simulink model "Quadcopter_nonlinear_LQR"  (R2020a)
settings: Solver=ode4  StartTime=0.0  StopTime=15  FixedStep=0.01  RelTol=1e-3
InitFcn:
  | linear_LQR_riccati_solver
values from neighbouring files (symbols this model uses):
  A1 = (h_cg * g * m_tot) / (m_tot * h_cg^2 + J_xx)    [QuadConstants.m]
  A2 = (2*m_tot * h_cg^2 + J_yy -J_zz) / (m_tot * h_cg^2 + J_xx)    [QuadConstants.m]
  A3 = (b * d_cg) / (m_tot * h_cg^2 + J_xx)    [QuadConstants.m]
  A4 = (J_R) / (m_tot * h_cg^2 + J_xx)    [QuadConstants.m]
  A5 = (m1 * g * miu_k * r_x) / (m_tot * h_cg^2 + J_xx)    [QuadConstants.m]
  B1 = (h_cg * g * m_tot) / (m_tot * h_cg^2 + J_yy)    [QuadConstants.m]
  B2 = (-2*m_tot * h_cg^2 - J_xx + J_zz) / (m_tot * h_cg^2 + J_yy)    [QuadConstants.m]
  B3 = (b * d_cg) / (m_tot * h_cg^2 + J_yy)    [QuadConstants.m]
  B4 = (-J_R) / (m_tot * h_cg^2 + J_yy)    [QuadConstants.m]
  B5 = (m2 * g * miu_k * r_y) / (m_tot * h_cg^2 + J_yy)    [QuadConstants.m]
  C1 = (J_xx - J_yy) / (J_zz)    [QuadConstants.m]
  C2 = (d) / (J_zz)    [QuadConstants.m]
  C3 = (m3 * g * miu_k * r_z) / (J_zz)    [QuadConstants.m]
undefined symbols (not defined in the file or in its folder): LQR_feedback_gain, magnitude, x0
settings Model: Creator=Ali  LastModifiedBy=Ali

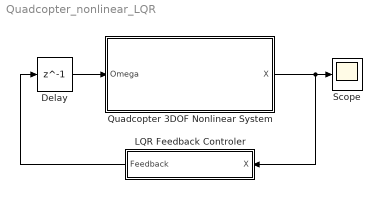
== system Quadcopter_nonlinear_LQR ==
  Delay : Delay  DelayLength=1
  LQR Feedback Controler : Subsystem
  Quadcopter 3DOF Nonlinear System : Subsystem  TreatAsAtomicUnit=on
  Scope : Scope
  wires:
  Quadcopter 3DOF Nonlinear System/1(X) -> LQR Feedback Controler/1(X), Scope/1
  LQR Feedback Controler/1(Feedback) -> Delay/1
  Delay/1 -> Quadcopter 3DOF Nonlinear System/1(Omega)

== system Quadcopter_nonlinear_LQR/LQR Feedback Controler ==
  X : Inport
  Add : Sum
  Constant : Constant  Value=LQR_feedback_gain
  Constant1 : Constant  Value=2000
  Product : Product  Multiplication=Matrix(*)
  Feedback : Outport
  wires:
  X/1 -> Product/2
  Constant/1 -> Product/1
  Product/1 -> Add/2
  Constant1/1 -> Add/1
  Add/1 -> Feedback/1

== system Quadcopter_nonlinear_LQR/Quadcopter 3DOF Nonlinear System ==
  Omega : Inport
  Integrator : Integrator  InitialCondition=x0
  Quad System : Subsystem
  X : Outport
  wires:
  Integrator/1 -> Quad System/1(X), X/1  "X"
  Quad System/1(dot(X)) -> Integrator/1  "dot(X)"
  Omega/1 -> Quad System/2(Omega)

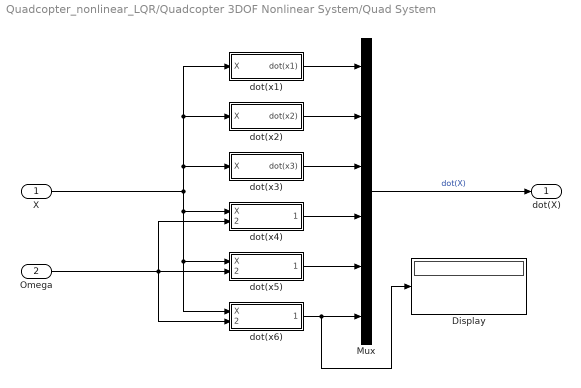
== system Quadcopter_nonlinear_LQR/Quadcopter 3DOF Nonlinear System/Quad System ==
  X : Inport
  Omega : Inport  Port=2
  Display : Display
  Mux : Mux  Inputs=6
  dot(x1) : Subsystem
  dot(x2) : Subsystem
  dot(x3) : Subsystem
  dot(x4) : Subsystem
  dot(x5) : Subsystem
  dot(x6) : Subsystem
  dot(X) : Outport
  wires:
  Mux/1 -> dot(X)/1  "dot(X)"
  X/1 -> dot(x1)/1(X), dot(x2)/1(X), dot(x3)/1(X), dot(x6)/1(X), dot(x5)/1(X), dot(x4)/1(X)
  Omega/1 -> dot(x4)/2(Omega), dot(x6)/2(Omega), dot(x5)/2(Omega)
  dot(x5)/1(dot(x5)) -> Mux/5
  dot(x2)/1(dot(x2)) -> Mux/2
  dot(x4)/1(dot(x4)) -> Mux/4
  dot(x3)/1(dot(x3)) -> Mux/3
  dot(x1)/1(dot(x1)) -> Mux/1
  dot(x6)/1(dot(x6)) -> Display/1, Mux/6

== system Quadcopter_nonlinear_LQR/Quadcopter 3DOF Nonlinear System/Quad System/dot(x1) ==
  X : Inport
  1 : Subsystem
  Add : Sum  Inputs=+++
  Subsystem : Subsystem
  Subsystem1 : Subsystem
  dot(x1) : Outport
  wires:
  X/1 -> Subsystem1/1(X), Subsystem/1(X), 1/1(X)  "X"
  Subsystem1/1(x4) -> Add/3
  Subsystem/1(x6cos(x1)tan(x2)) -> Add/2
  Add/1 -> dot(x1)/1
  1/1(x5sin(x1)tan(x2)) -> Add/1

== system Quadcopter_nonlinear_LQR/Quadcopter 3DOF Nonlinear System/Quad System/dot(x2) ==
  X : Inport
  1 : Subsystem
  Add : Sum  Inputs=+-
  Subsystem : Subsystem
  dot(x2) : Outport
  wires:
  X/1 -> 1/1(X), Subsystem/1(X)  "X"
  Subsystem/1(x6sin(x1)) -> Add/2
  Add/1 -> dot(x2)/1
  1/1(x5cos(x1)) -> Add/1

== system Quadcopter_nonlinear_LQR/Quadcopter 3DOF Nonlinear System/Quad System/dot(x3) ==
  X : Inport
  1 : Subsystem
  Add : Sum
  Product : Product
  Subsystem : Subsystem
  Subsystem1 : Subsystem
  dot(x3) : Outport
  wires:
  X/1 -> Subsystem1/1(X), Subsystem/1(X), 1/1(X)  "X"
  Subsystem/1(x6cos(x1)) -> Add/2
  1/1(x5sin(x1)) -> Add/1
  Product/1 -> dot(x3)/1
  Add/1 -> Product/1
  Subsystem1/1(sec(x2)) -> Product/2

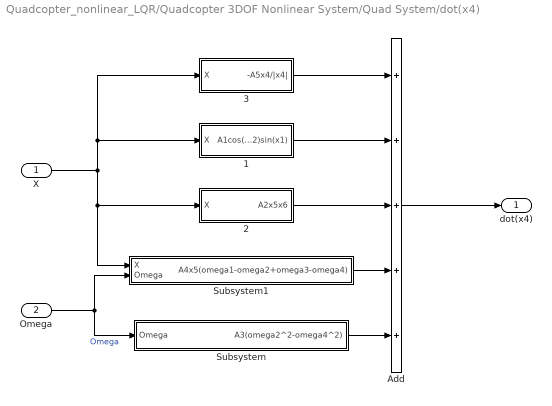
== system Quadcopter_nonlinear_LQR/Quadcopter 3DOF Nonlinear System/Quad System/dot(x4) ==
  X : Inport
  Omega : Inport  Port=2
  1 : Subsystem
  2 : Subsystem
  3 : Subsystem
  Add : Sum  Inputs=+++++
  Subsystem : Subsystem
  Subsystem1 : Subsystem
  dot(x4) : Outport
  wires:
  X/1 -> Subsystem1/1(X), 2/1(X), 3/1(X), 1/1(X)
  Omega/1 -> Subsystem1/2(Omega), Subsystem/1(Omega)  "Omega"
  Add/1 -> dot(x4)/1
  3/1("-A5x4/|x4| ") -> Add/1
  1/1(A1cos(x2)sin(x1)) -> Add/2
  2/1(A2x5x6) -> Add/3
  Subsystem1/1(A4x5(omega1-omega2+omega3-omega4)) -> Add/4
  Subsystem/1(A3(omega2^2-omega4^2)) -> Add/5

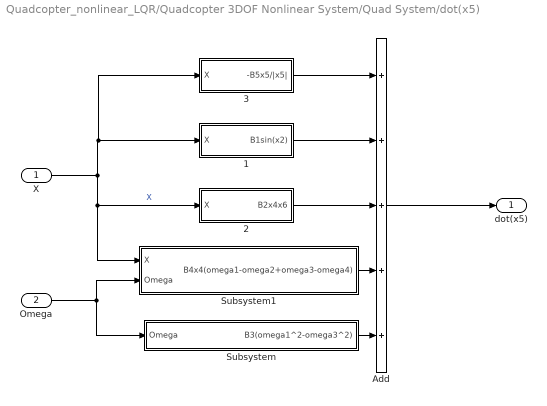
== system Quadcopter_nonlinear_LQR/Quadcopter 3DOF Nonlinear System/Quad System/dot(x5) ==
  X : Inport
  Omega : Inport  Port=2
  1 : Subsystem
  2 : Subsystem
  3 : Subsystem
  Add : Sum  Inputs=+++++
  Subsystem : Subsystem
  Subsystem1 : Subsystem
  dot(x5) : Outport
  wires:
  X/1 -> Subsystem1/1(X), 2/1(X), 3/1(X), 1/1(X)  "X"
  Omega/1 -> Subsystem/1(Omega), Subsystem1/2(Omega)
  Add/1 -> dot(x5)/1
  3/1("-B5x5/|x5| ") -> Add/1
  1/1(B1sin(x2)) -> Add/2
  2/1(B2x4x6) -> Add/3
  Subsystem1/1(B4x4(omega1-omega2+omega3-omega4)) -> Add/4
  Subsystem/1(B3(omega1^2-omega3^2)) -> Add/5

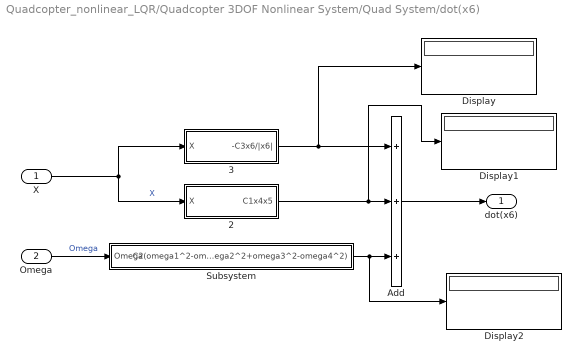
== system Quadcopter_nonlinear_LQR/Quadcopter 3DOF Nonlinear System/Quad System/dot(x6) ==
  X : Inport
  Omega : Inport  Port=2
  2 : Subsystem
  3 : Subsystem
  Add : Sum  Inputs=+++
  Display : Display
  Display1 : Display
  Display2 : Display
  Subsystem : Subsystem
  dot(x6) : Outport
  wires:
  Omega/1 -> Subsystem/1(Omega)  "Omega"
  Add/1 -> dot(x6)/1
  3/1("-C3x6/|x6| ") -> Display/1, Add/1
  2/1(C1x4x5) -> Display1/1, Add/2
  Subsystem/1(C2(omega1^2-omega2^2+omega3^2-omega4^2)) -> Display2/1, Add/3
  X/1 -> 3/1(X), 2/1(X)  "X"

== system Quadcopter_nonlinear_LQR/Quadcopter 3DOF Nonlinear System/Quad System/dot(x1)/1 ==
  X : Inport
  Demux : Demux  Outputs=6
  Subsystem : Subsystem
  Terminator : Terminator
  Terminator1 : Terminator
  Terminator2 : Terminator
  x5sin(x1)tan(x2) : Outport
  wires:
  Demux/2 -> Subsystem/2(x2)  "x2"
  Demux/4 -> Terminator1/1  "x4"
  X/1 -> Demux/1  "x"
  Demux/1 -> Subsystem/1(x1)  "x1"
  Demux/3 -> Terminator/1  "x3"
  Demux/6 -> Terminator2/1  "x6"
  Demux/5 -> Subsystem/3(x5)  "x5"
  Subsystem/1(x5sin(x1)tan(x2)) -> x5sin(x1)tan(x2)/1

== system Quadcopter_nonlinear_LQR/Quadcopter 3DOF Nonlinear System/Quad System/dot(x1)/Subsystem ==
  X : Inport
  Demux : Demux  Outputs=6
  Subsystem1 : Subsystem
  Terminator : Terminator
  Terminator1 : Terminator
  Terminator3 : Terminator
  x6cos(x1)tan(x2) : Outport
  wires:
  Demux/1 -> Subsystem1/1(x1)  "x1"
  Demux/3 -> Terminator/1  "x3"
  Demux/4 -> Terminator1/1  "x4"
  Demux/5 -> Terminator3/1  "x5"
  Demux/6 -> Subsystem1/3(x6)  "x6"
  Subsystem1/1(x6cos(x1)tan(x2)) -> x6cos(x1)tan(x2)/1  "x6cos(x1)tan(x2)"
  X/1 -> Demux/1  "X"
  Demux/2 -> Subsystem1/2(x2)  "x2"

== system Quadcopter_nonlinear_LQR/Quadcopter 3DOF Nonlinear System/Quad System/dot(x1)/Subsystem1 ==
  X : Inport
  Demux : Demux  Outputs=6
  Terminator{,2..5} (5 alike) : Terminator
  x4 : Outport
  wires:
  Demux/6 -> Terminator5/1  "x6"
  X/1 -> Demux/1
  Demux/3 -> Terminator/1  "x3"
  Demux/1 -> Terminator4/1  "x1"
  Demux/2 -> Terminator2/1  "x2"
  Demux/5 -> Terminator3/1  "x5"
  Demux/4 -> x4/1  "x4"

== system Quadcopter_nonlinear_LQR/Quadcopter 3DOF Nonlinear System/Quad System/dot(x2)/1 ==
  X : Inport
  Demux : Demux  Outputs=6
  Subsystem : Subsystem
  Terminator{,1..3} (4 alike) : Terminator
  x5cos(x1) : Outport
  wires:
  Demux/4 -> Terminator1/1  "x4"
  X/1 -> Demux/1  "x"
  Demux/1 -> Subsystem/1(x1)  "x1"
  Demux/3 -> Terminator/1  "x3"
  Demux/6 -> Terminator2/1  "x6"
  Demux/5 -> Subsystem/2(x5)  "x5"
  Subsystem/1(Out1) -> x5cos(x1)/1
  Demux/2 -> Terminator3/1  "x2"

== system Quadcopter_nonlinear_LQR/Quadcopter 3DOF Nonlinear System/Quad System/dot(x2)/Subsystem ==
  X : Inport
  Demux : Demux  Outputs=6
  Subsystem1 : Subsystem
  Terminator{,1..3} (4 alike) : Terminator
  x6sin(x1) : Outport
  wires:
  Demux/1 -> Subsystem1/1(x1)  "x1"
  Demux/3 -> Terminator/1  "x3"
  Demux/4 -> Terminator1/1  "x4"
  Demux/5 -> Terminator3/1  "x5"
  Demux/6 -> Subsystem1/2(x6)  "x6"
  Subsystem1/1(Out1) -> x6sin(x1)/1  "x6sin(x1)"
  X/1 -> Demux/1  "X"
  Demux/2 -> Terminator2/1  "x2"

== system Quadcopter_nonlinear_LQR/Quadcopter 3DOF Nonlinear System/Quad System/dot(x3)/1 ==
  X : Inport
  Demux : Demux  Outputs=6
  Subsystem : Subsystem
  Terminator{,1..3} (4 alike) : Terminator
  x5sin(x1) : Outport
  wires:
  Demux/4 -> Terminator1/1  "x4"
  X/1 -> Demux/1  "x"
  Demux/1 -> Subsystem/1(x1)  "x1"
  Demux/3 -> Terminator/1  "x3"
  Demux/6 -> Terminator2/1  "x6"
  Demux/5 -> Subsystem/2(x5)  "x5"
  Subsystem/1(x5sin(x1)) -> x5sin(x1)/1
  Demux/2 -> Terminator3/1  "x2"

== system Quadcopter_nonlinear_LQR/Quadcopter 3DOF Nonlinear System/Quad System/dot(x3)/Subsystem ==
  X : Inport
  Demux : Demux  Outputs=6
  Subsystem1 : Subsystem
  Terminator{,1..3} (4 alike) : Terminator
  x6cos(x1) : Outport
  wires:
  Demux/1 -> Subsystem1/1(x1)  "x1"
  Demux/3 -> Terminator/1  "x3"
  Demux/4 -> Terminator1/1  "x4"
  Demux/5 -> Terminator3/1  "x5"
  Demux/6 -> Subsystem1/2(x6)  "x6"
  Subsystem1/1(Out1) -> x6cos(x1)/1  "x6cos(x1)"
  X/1 -> Demux/1  "X"
  Demux/2 -> Terminator2/1  "x2"

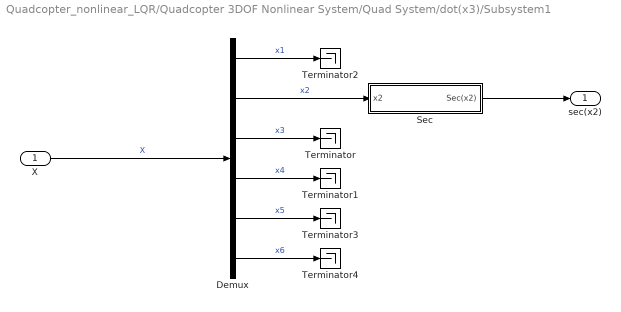
== system Quadcopter_nonlinear_LQR/Quadcopter 3DOF Nonlinear System/Quad System/dot(x3)/Subsystem1 ==
  X : Inport
  Demux : Demux  Outputs=6
  Sec : Subsystem
  Terminator{,1..4} (5 alike) : Terminator
  sec(x2) : Outport
  wires:
  Demux/3 -> Terminator/1  "x3"
  Demux/4 -> Terminator1/1  "x4"
  Demux/5 -> Terminator3/1  "x5"
  X/1 -> Demux/1  "X"
  Demux/1 -> Terminator2/1  "x1"
  Demux/6 -> Terminator4/1  "x6"
  Demux/2 -> Sec/1(x2)  "x2"
  Sec/1(Sec(x2)) -> sec(x2)/1

== system Quadcopter_nonlinear_LQR/Quadcopter 3DOF Nonlinear System/Quad System/dot(x4)/1 ==
  X : Inport
  Demux : Demux  Outputs=6
  Subsystem : Subsystem
  Terminator{,1..3} (4 alike) : Terminator
  A1cos(x2)sin(x1) : Outport
  wires:
  Demux/4 -> Terminator1/1  "x4"
  X/1 -> Demux/1  "x"
  Demux/1 -> Subsystem/1(x1)  "x1"
  Demux/3 -> Terminator/1  "x3"
  Demux/6 -> Terminator2/1  "x6"
  Subsystem/1(A1cos(x2)sin(x1)) -> A1cos(x2)sin(x1)/1
  Demux/2 -> Subsystem/2(x2)  "x2"
  Demux/5 -> Terminator3/1  "x5"

== system Quadcopter_nonlinear_LQR/Quadcopter 3DOF Nonlinear System/Quad System/dot(x4)/2 ==
  X : Inport
  Demux : Demux  Outputs=6
  Subsystem : Subsystem
  Terminator{,1,4..5} (4 alike) : Terminator
  A2x5x6 : Outport
  wires:
  Demux/4 -> Terminator1/1  "x4"
  X/1 -> Demux/1  "x"
  Demux/3 -> Terminator/1  "x3"
  Demux/6 -> Subsystem/2(x6)  "x6"
  Subsystem/1(A2x5x6) -> A2x5x6/1
  Demux/5 -> Subsystem/1(x5)  "x5"
  Demux/1 -> Terminator4/1  "x1"
  Demux/2 -> Terminator5/1  "x2"

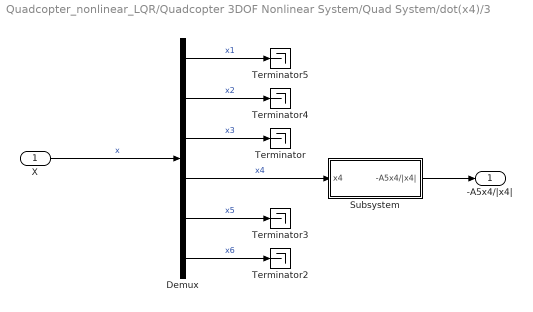
== system Quadcopter_nonlinear_LQR/Quadcopter 3DOF Nonlinear System/Quad System/dot(x4)/3 ==
  X : Inport
  Demux : Demux  Outputs=6
  Subsystem : Subsystem
  Terminator{,2..5} (5 alike) : Terminator
  "-A5x4/|x4| " : Outport
  wires:
  X/1 -> Demux/1  "x"
  Demux/1 -> Terminator5/1  "x1"
  Demux/3 -> Terminator/1  "x3"
  Demux/6 -> Terminator2/1  "x6"
  Demux/2 -> Terminator4/1  "x2"
  Demux/5 -> Terminator3/1  "x5"
  Demux/4 -> Subsystem/1(x4)  "x4"
  Subsystem/1("-A5x4/|x4| ") -> "-A5x4/|x4| "/1

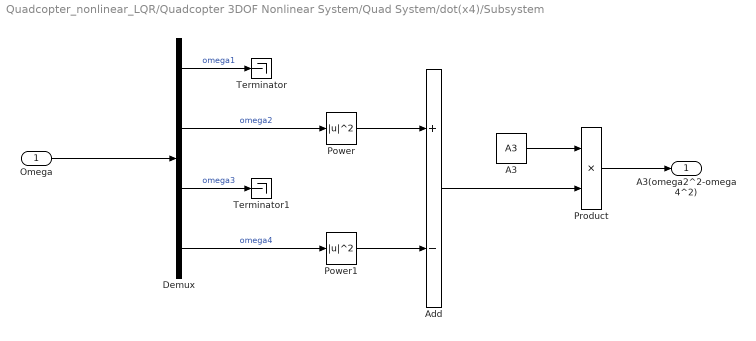
== system Quadcopter_nonlinear_LQR/Quadcopter 3DOF Nonlinear System/Quad System/dot(x4)/Subsystem ==
  Omega : Inport
  A3 : Constant  Value=A3
  Add : Sum  Inputs=+-
  Demux : Demux
  Power : Math  Operator=magnitude^2  SaturateOnIntegerOverflow=on
  Power1 : Math  Operator=magnitude^2  SaturateOnIntegerOverflow=on
  Product : Product
  Terminator : Terminator
  Terminator1 : Terminator
  A3(omega2^2-omega4^2) : Outport
  wires:
  Product/1 -> A3(omega2^2-omega4^2)/1
  Power1/1 -> Add/2
  Demux/2 -> Power/1  "omega2"
  Demux/4 -> Power1/1  "omega4"
  Add/1 -> Product/2
  Power/1 -> Add/1
  A3/1 -> Product/1
  Omega/1 -> Demux/1
  Demux/3 -> Terminator1/1  "omega3"
  Demux/1 -> Terminator/1  "omega1"

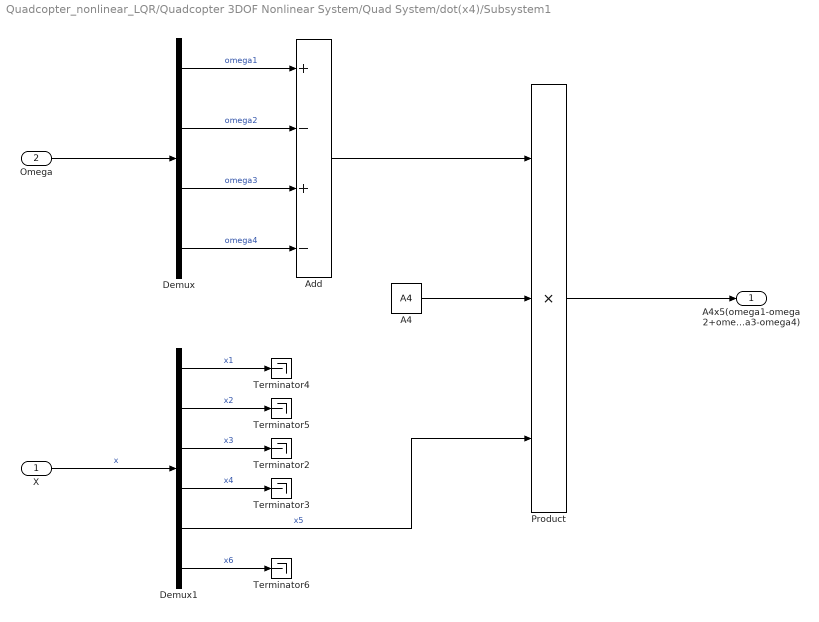
== system Quadcopter_nonlinear_LQR/Quadcopter 3DOF Nonlinear System/Quad System/dot(x4)/Subsystem1 ==
  X : Inport
  Omega : Inport  Port=2
  A4 : Constant  Value=A4
  Add : Sum  Inputs=+-+-
  Demux : Demux
  Demux1 : Demux  Outputs=6
  Product : Product  Inputs=3
  Terminator{2..6} (5 alike) : Terminator
  A4x5(omega1-omega2+omega3-omega4) : Outport
  wires:
  Omega/1 -> Demux/1
  Demux1/6 -> Terminator6/1  "x6"
  Demux1/5 -> Product/3  "x5"
  X/1 -> Demux1/1  "x"
  Demux1/2 -> Terminator5/1  "x2"
  Demux1/3 -> Terminator2/1  "x3"
  Demux1/4 -> Terminator3/1  "x4"
  Demux1/1 -> Terminator4/1  "x1"
  Demux/1 -> Add/1  "omega1"
  Demux/2 -> Add/2  "omega2"
  Demux/3 -> Add/3  "omega3"
  Demux/4 -> Add/4  "omega4"
  Add/1 -> Product/1
  A4/1 -> Product/2
  Product/1 -> A4x5(omega1-omega2+omega3-omega4)/1

== system Quadcopter_nonlinear_LQR/Quadcopter 3DOF Nonlinear System/Quad System/dot(x5)/1 ==
  X : Inport
  Demux : Demux  Outputs=6
  Subsystem : Subsystem
  Terminator{,1..4} (5 alike) : Terminator
  B1sin(x2) : Outport
  wires:
  Demux/4 -> Terminator1/1  "x4"
  X/1 -> Demux/1  "x"
  Demux/3 -> Terminator/1  "x3"
  Demux/6 -> Terminator2/1  "x6"
  Subsystem/1(B1sin(x2)) -> B1sin(x2)/1
  Demux/2 -> Subsystem/1(x2)  "x2"
  Demux/5 -> Terminator3/1  "x5"
  Demux/1 -> Terminator4/1  "x1"

== system Quadcopter_nonlinear_LQR/Quadcopter 3DOF Nonlinear System/Quad System/dot(x5)/2 ==
  X : Inport
  Demux : Demux  Outputs=6
  Subsystem : Subsystem
  Terminator{,2,4..5} (4 alike) : Terminator
  B2x4x6 : Outport
  wires:
  Demux/4 -> Subsystem/1(x4)  "x4"
  X/1 -> Demux/1  "x"
  Demux/3 -> Terminator/1  "x3"
  Demux/6 -> Subsystem/2(x6)  "x6"
  Subsystem/1(B2x4x6) -> B2x4x6/1
  Demux/1 -> Terminator4/1  "x1"
  Demux/2 -> Terminator5/1  "x2"
  Demux/5 -> Terminator2/1  "x5"

== system Quadcopter_nonlinear_LQR/Quadcopter 3DOF Nonlinear System/Quad System/dot(x5)/3 ==
  X : Inport
  Demux : Demux  Outputs=6
  Subsystem : Subsystem
  Terminator{,1..2,4..5} (5 alike) : Terminator
  "-B5x5/|x5| " : Outport
  wires:
  X/1 -> Demux/1  "x"
  Demux/1 -> Terminator5/1  "x1"
  Demux/3 -> Terminator/1  "x3"
  Demux/6 -> Terminator2/1  "x6"
  Demux/2 -> Terminator4/1  "x2"
  Demux/5 -> Subsystem/1(x5)  "x5"
  Subsystem/1("-B5x5/|x5| ") -> "-B5x5/|x5| "/1
  Demux/4 -> Terminator1/1  "x4"

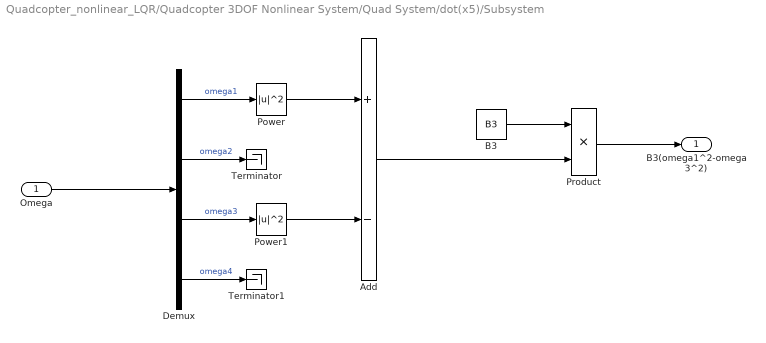
== system Quadcopter_nonlinear_LQR/Quadcopter 3DOF Nonlinear System/Quad System/dot(x5)/Subsystem ==
  Omega : Inport
  Add : Sum  Inputs=+-
  B3 : Constant  Value=B3
  Demux : Demux
  Power : Math  Operator=magnitude^2  SaturateOnIntegerOverflow=on
  Power1 : Math  Operator=magnitude^2  SaturateOnIntegerOverflow=on
  Product : Product
  Terminator : Terminator
  Terminator1 : Terminator
  B3(omega1^2-omega3^2) : Outport
  wires:
  Product/1 -> B3(omega1^2-omega3^2)/1
  Power1/1 -> Add/2
  Add/1 -> Product/2
  Power/1 -> Add/1
  B3/1 -> Product/1
  Omega/1 -> Demux/1
  Demux/3 -> Power1/1  "omega3"
  Demux/1 -> Power/1  "omega1"
  Demux/2 -> Terminator/1  "omega2"
  Demux/4 -> Terminator1/1  "omega4"

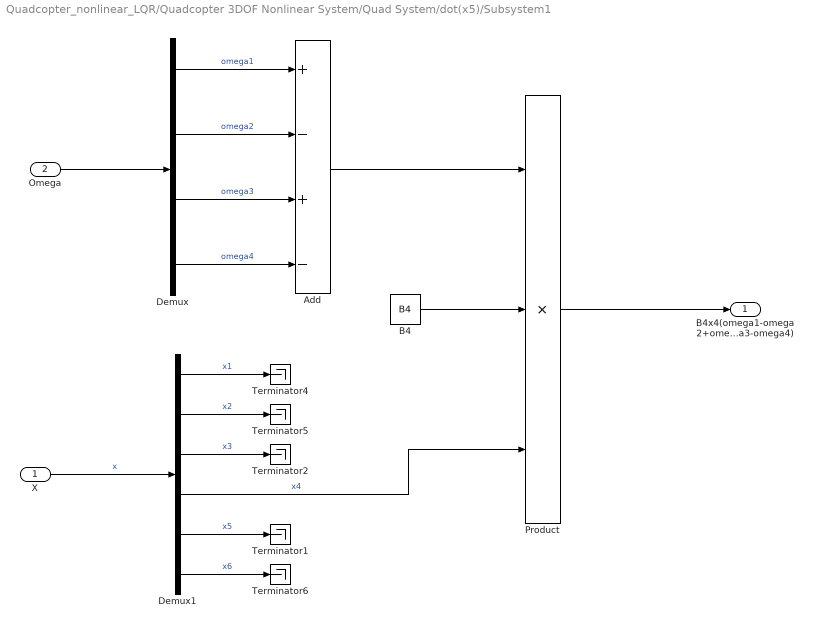
== system Quadcopter_nonlinear_LQR/Quadcopter 3DOF Nonlinear System/Quad System/dot(x5)/Subsystem1 ==
  X : Inport
  Omega : Inport  Port=2
  Add : Sum  Inputs=+-+-
  B4 : Constant  Value=B4
  Demux : Demux
  Demux1 : Demux  Outputs=6
  Product : Product  Inputs=3
  Terminator{1..2,4..6} (5 alike) : Terminator
  B4x4(omega1-omega2+omega3-omega4) : Outport
  wires:
  Omega/1 -> Demux/1
  Demux1/6 -> Terminator6/1  "x6"
  X/1 -> Demux1/1  "x"
  Demux1/2 -> Terminator5/1  "x2"
  Demux1/3 -> Terminator2/1  "x3"
  Demux1/4 -> Product/3  "x4"
  Demux1/1 -> Terminator4/1  "x1"
  Demux/1 -> Add/1  "omega1"
  Demux/2 -> Add/2  "omega2"
  Demux/3 -> Add/3  "omega3"
  Demux/4 -> Add/4  "omega4"
  Add/1 -> Product/1
  B4/1 -> Product/2
  Product/1 -> B4x4(omega1-omega2+omega3-omega4)/1
  Demux1/5 -> Terminator1/1  "x5"

== system Quadcopter_nonlinear_LQR/Quadcopter 3DOF Nonlinear System/Quad System/dot(x6)/2 ==
  X : Inport
  Demux : Demux  Outputs=6
  Subsystem : Subsystem
  Terminator{,2,4..5} (4 alike) : Terminator
  C1x4x5 : Outport
  wires:
  Demux/4 -> Subsystem/1(x4)  "x4"
  X/1 -> Demux/1  "x"
  Demux/3 -> Terminator/1  "x3"
  Subsystem/1(C1x4x5) -> C1x4x5/1
  Demux/1 -> Terminator4/1  "x1"
  Demux/2 -> Terminator5/1  "x2"
  Demux/5 -> Subsystem/2(x5)  "x5"
  Demux/6 -> Terminator2/1  "x6"

== system Quadcopter_nonlinear_LQR/Quadcopter 3DOF Nonlinear System/Quad System/dot(x6)/3 ==
  X : Inport
  Demux : Demux  Outputs=6
  Subsystem : Subsystem
  Terminator{,1,3..5} (5 alike) : Terminator
  "-C3x6/|x6| " : Outport
  wires:
  X/1 -> Demux/1  "x"
  Demux/1 -> Terminator5/1  "x1"
  Demux/3 -> Terminator/1  "x3"
  Demux/6 -> Subsystem/1(x6)  "x6"
  Demux/2 -> Terminator4/1  "x2"
  Demux/5 -> Terminator3/1  "x5"
  Subsystem/1("-C3x6/|x6| ") -> "-C3x6/|x6| "/1
  Demux/4 -> Terminator1/1  "x4"

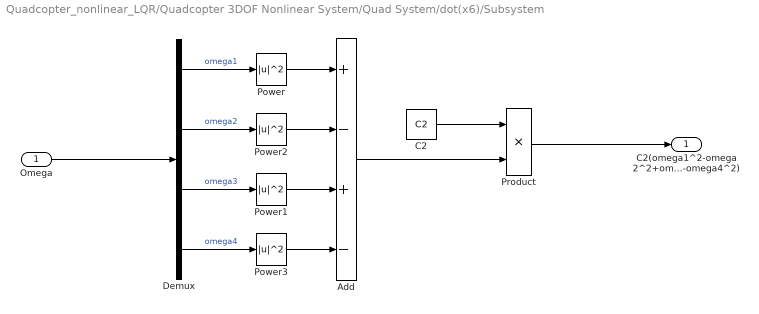
== system Quadcopter_nonlinear_LQR/Quadcopter 3DOF Nonlinear System/Quad System/dot(x6)/Subsystem ==
  Omega : Inport
  Add : Sum  Inputs=+-+-
  C2 : Constant  Value=C2
  Demux : Demux
  Power{,1..3} (4 alike) : Math  Operator=magnitude^2  SaturateOnIntegerOverflow=on
  Product : Product
  C2(omega1^2-omega2^2+omega3^2-omega4^2) : Outport
  wires:
  Omega/1 -> Demux/1
  Demux/3 -> Power1/1  "omega3"
  Demux/1 -> Power/1  "omega1"
  Demux/2 -> Power2/1  "omega2"
  Demux/4 -> Power3/1  "omega4"
  C2/1 -> Product/1
  Add/1 -> Product/2
  Product/1 -> C2(omega1^2-omega2^2+omega3^2-omega4^2)/1
  Power/1 -> Add/1
  Power2/1 -> Add/2
  Power1/1 -> Add/3
  Power3/1 -> Add/4

== system Quadcopter_nonlinear_LQR/Quadcopter 3DOF Nonlinear System/Quad System/dot(x1)/1/Subsystem ==
  x1 : Inport
  x2 : Inport  Port=2
  x5 : Inport  Port=3
  Product : Product  Inputs=3
  Sin : Trigonometry
  Tan : Trigonometry  Operator=tan
  x5sin(x1)tan(x2) : Outport
  wires:
  Sin/1 -> Product/1
  x5/1 -> Product/3
  Product/1 -> x5sin(x1)tan(x2)/1
  x1/1 -> Sin/1
  x2/1 -> Tan/1
  Tan/1 -> Product/2

== system Quadcopter_nonlinear_LQR/Quadcopter 3DOF Nonlinear System/Quad System/dot(x1)/Subsystem/Subsystem1 ==
  x1 : Inport
  x2 : Inport  Port=2
  x6 : Inport  Port=3
  Cos : Trigonometry  Operator=cos
  Product1 : Product  Inputs=3
  Tan : Trigonometry  Operator=tan
  x6cos(x1)tan(x2) : Outport
  wires:
  x6/1 -> Product1/3
  x1/1 -> Cos/1
  Cos/1 -> Product1/1
  x2/1 -> Tan/1
  Product1/1 -> x6cos(x1)tan(x2)/1
  Tan/1 -> Product1/2

== system Quadcopter_nonlinear_LQR/Quadcopter 3DOF Nonlinear System/Quad System/dot(x2)/1/Subsystem ==
  x1 : Inport
  x5 : Inport  Port=2
  Cos : Trigonometry  Operator=cos
  Product : Product
  Out1 : Outport
  wires:
  Cos/1 -> Product/1
  Product/1 -> Out1/1
  x1/1 -> Cos/1
  x5/1 -> Product/2

== system Quadcopter_nonlinear_LQR/Quadcopter 3DOF Nonlinear System/Quad System/dot(x2)/Subsystem/Subsystem1 ==
  x1 : Inport
  x6 : Inport  Port=2
  Product1 : Product
  Sin : Trigonometry
  Out1 : Outport
  wires:
  x6/1 -> Product1/2
  x1/1 -> Sin/1
  Sin/1 -> Product1/1
  Product1/1 -> Out1/1

== system Quadcopter_nonlinear_LQR/Quadcopter 3DOF Nonlinear System/Quad System/dot(x3)/1/Subsystem ==
  x1 : Inport
  x5 : Inport  Port=2
  Product : Product
  Sin : Trigonometry
  x5sin(x1) : Outport
  wires:
  Sin/1 -> Product/1
  Product/1 -> x5sin(x1)/1
  x1/1 -> Sin/1
  x5/1 -> Product/2

== system Quadcopter_nonlinear_LQR/Quadcopter 3DOF Nonlinear System/Quad System/dot(x3)/Subsystem/Subsystem1 ==
  x1 : Inport
  x6 : Inport  Port=2
  Cos : Trigonometry  Operator=cos
  Product1 : Product
  Out1 : Outport
  wires:
  x6/1 -> Product1/2
  x1/1 -> Cos/1
  Cos/1 -> Product1/1
  Product1/1 -> Out1/1

== system Quadcopter_nonlinear_LQR/Quadcopter 3DOF Nonlinear System/Quad System/dot(x3)/Subsystem1/Sec ==
  x2 : Inport
  Constant : Constant
  Cos : Trigonometry  Operator=cos
  Divide : Product  Inputs=*/
  Sec(x2) : Outport
  wires:
  Constant/1 -> Divide/1
  Cos/1 -> Divide/2
  Divide/1 -> Sec(x2)/1
  x2/1 -> Cos/1

== system Quadcopter_nonlinear_LQR/Quadcopter 3DOF Nonlinear System/Quad System/dot(x4)/1/Subsystem ==
  x1 : Inport
  x2 : Inport  Port=2
  A1 : Constant  Value=A1
  Cos : Trigonometry  Operator=cos
  Product : Product  Inputs=3
  Sin : Trigonometry
  A1cos(x2)sin(x1) : Outport
  wires:
  Sin/1 -> Product/1
  Product/1 -> A1cos(x2)sin(x1)/1
  x1/1 -> Sin/1
  x2/1 -> Cos/1
  Cos/1 -> Product/2
  A1/1 -> Product/3

== system Quadcopter_nonlinear_LQR/Quadcopter 3DOF Nonlinear System/Quad System/dot(x4)/2/Subsystem ==
  x5 : Inport
  x6 : Inport  Port=2
  A2 : Constant  Value=A2
  Product : Product  Inputs=3
  A2x5x6 : Outport
  wires:
  x5/1 -> Product/1
  Product/1 -> A2x5x6/1
  x6/1 -> Product/2
  A2/1 -> Product/3

== system Quadcopter_nonlinear_LQR/Quadcopter 3DOF Nonlinear System/Quad System/dot(x4)/3/Subsystem ==
  x4 : Inport
  A5 : Constant  Value=A5
  Gain : Gain  Gain=-1
  Switch : Switch  Criteria=u2 > Threshold
  "-A5x4/|x4| " : Outport
  wires:
  Switch/1 -> "-A5x4/|x4| "/1
  A5/1 -> Switch/3, Gain/1
  x4/1 -> Switch/2
  Gain/1 -> Switch/1

== system Quadcopter_nonlinear_LQR/Quadcopter 3DOF Nonlinear System/Quad System/dot(x5)/1/Subsystem ==
  x2 : Inport
  B1 : Constant  Value=B1
  Product : Product
  Sin : Trigonometry
  B1sin(x2) : Outport
  wires:
  Product/1 -> B1sin(x2)/1
  x2/1 -> Sin/1
  B1/1 -> Product/2
  Sin/1 -> Product/1

== system Quadcopter_nonlinear_LQR/Quadcopter 3DOF Nonlinear System/Quad System/dot(x5)/2/Subsystem ==
  x4 : Inport
  x6 : Inport  Port=2
  B2 : Constant  Value=B2
  Product : Product  Inputs=3
  B2x4x6 : Outport
  wires:
  x4/1 -> Product/1
  Product/1 -> B2x4x6/1
  x6/1 -> Product/2
  B2/1 -> Product/3

== system Quadcopter_nonlinear_LQR/Quadcopter 3DOF Nonlinear System/Quad System/dot(x5)/3/Subsystem ==
  x5 : Inport
  B5 : Constant  Value=B5
  Gain : Gain  Gain=-1
  Switch : Switch  Criteria=u2 > Threshold
  "-B5x5/|x5| " : Outport
  wires:
  Switch/1 -> "-B5x5/|x5| "/1
  B5/1 -> Switch/3, Gain/1
  x5/1 -> Switch/2
  Gain/1 -> Switch/1

== system Quadcopter_nonlinear_LQR/Quadcopter 3DOF Nonlinear System/Quad System/dot(x6)/2/Subsystem ==
  x4 : Inport
  x5 : Inport  Port=2
  C1 : Constant  Value=C1
  Product : Product  Inputs=3
  C1x4x5 : Outport
  wires:
  x4/1 -> Product/1
  Product/1 -> C1x4x5/1
  x5/1 -> Product/2
  C1/1 -> Product/3

== system Quadcopter_nonlinear_LQR/Quadcopter 3DOF Nonlinear System/Quad System/dot(x6)/3/Subsystem ==
  x6 : Inport
  C3 : Constant  Value=C3
  Gain : Gain  Gain=-1
  Switch : Switch  Criteria=u2 > Threshold
  "-C3x6/|x6| " : Outport
  wires:
  Switch/1 -> "-C3x6/|x6| "/1
  C3/1 -> Switch/3, Gain/1
  x6/1 -> Switch/2
  Gain/1 -> Switch/1
